simulink model "matlab_control_demo_model_navigation"  (R2022b)
settings: Solver=FixedStepAuto  StartTime=0.0  StopTime=inf  RelTol=1e-3
values from neighbouring files (symbols this model uses):
  waypoints = [ ... (first row only)    [load_quadrotor_simulink_control_model_navigation.m]
libraries: slpidlib x10, sharedutil x2, sharedtransform x2, simulink x2, uavalgslib x1, simulink_extras x1
(part 1 of 2)
settings Model: PacingRate=0.100000  Creator=The MathWorks, Inc.  LastModifiedBy=v-zbraude
settings SolverCC: MaxZcPerStep=1
settings OptimizationCC: DefaultParameterBehavior=Inlined  EnhancedBackFolding=on  PassReuseOutputArgsAs=Individual arguments  ZeroExternalMemoryAtStartup=off  ZeroInternalMemoryAtStartup=off  MaxStackSize=64  OptimizeBlockOrder=speed  DifferentSizesBufferReuse=on  OptimizationCustomize=off  EfficientTunableParamExpr=on
settings DebuggingCC: ParameterTunabilityLossMsg=error
settings HardwareCC: ProdBitPerPointer=32  ProdBitPerSizeT=32  ProdBitPerPtrDiffT=32  ProdLargestAtomicInteger=Long  ProdLargestAtomicFloat=Double  ProdWordSize=32  ProdHWDeviceType=ARM Compatible->ARM Cortex
settings ModelReferenceCC: EnableRefExpFcnMdlSchedulingChecks=on
settings SFSimCC: MATLABDynamicMemAlloc=off
settings RTWCC: Description=Embedded Coder  SystemTargetFile=ert.tlc  TemplateMakefile=ert_default_tmf  Toolchain=GNU Tools for PX4 Autopilots  DLArmComputeVersion=19.05
settings CodeAppCC: ForceParamTrailComments=on  IgnoreCustomStorageClasses=off  MaxIdLength=63  OperatorAnnotations=on  SimulinkDataObjDesc=on  SFDataObjDesc=on  InsertBlockDesc=on
settings ERTTargetCC: ExtModeTransport=3  ExtModeStaticAlloc=on  ExtModeMexFile=ext_xcp  ExtModeIntrfLevel=Level2 - Open  ERTCustomFileTemplate=example_file_process.tlc

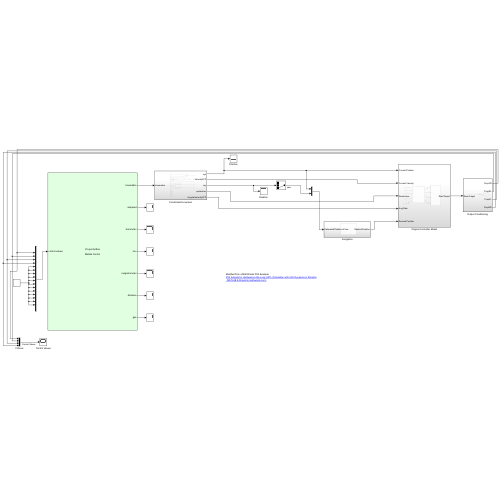
[thumbnail: Simulink's stored preview of the top-level diagram]
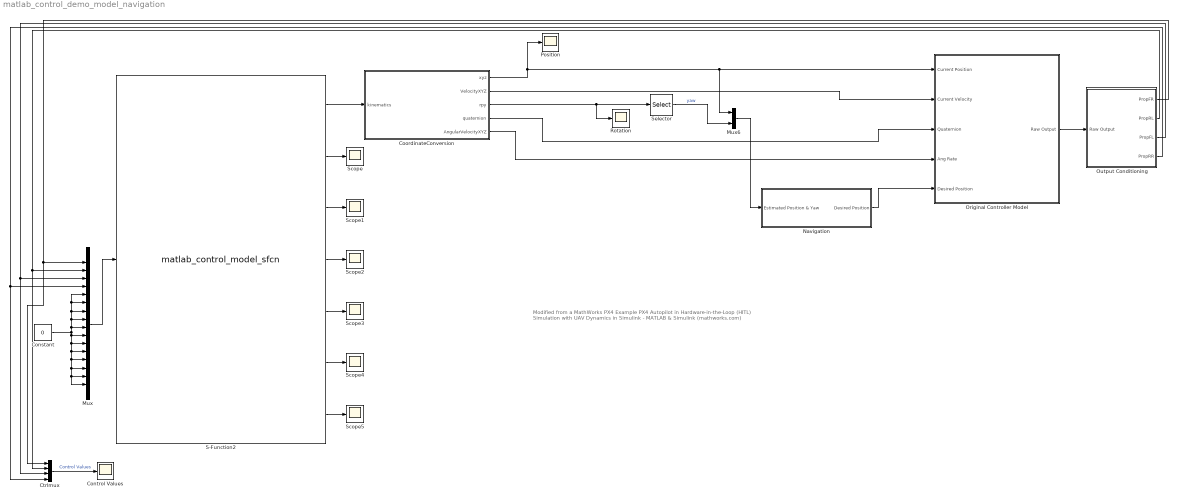
== system matlab_control_demo_model_navigation ==
  note: Modified from a MathWorks PX4 Example
      | PX4 Autopilot in Hardware-in-the-Loop (HITL) Simulation with UAV Dynamics in Simulink - MATLAB & Simulink (mathworks.com)
  Constant : Constant  Value=0
  Control Values : Scope
  CoordinateConversion : Subsystem
  Ctrlmux : Mux
  Mux : Mux  Inputs=16
  Mux6 : Mux  Inputs=2
  Navigation : Subsystem
  Original Controller Model : Subsystem
  Output Conditioning : Subsystem
  Position : Scope
  Rotation : Scope
  S-Function2 : S-Function  Priority=1  FunctionName=matlab_control_model_sfcn  Parameters=hostname,portnumber,timestep  SFunctionDeploymentMode=off  EnableBusSupport=off  mask{hostname=*, portnumber=8998, timestep=0.003}
      mask prompts: hostname "Host name:"; portnumber "Port number:"; timestep "AirSim time step:"
      mask Display:
      | disp("Project AirSim\n\n")
      | disp("\n\nMatlab Control")
      | port_label('input',1,'control values')
      | port_label('output',1,'kinematics')
      | port_label('output',2,'airspeed')
      | port_label('output',3,'barometer')
      | port_label('output',4,'imu')
      | port_label('output',5,'magnetometer')
      | port_label('output',6,'distance')
      | port_label('output',7,'gps')
  Scope{,1..5} (6 alike) : Scope
  Selector : Selector  InputPortWidth=3  IndexOptions=Index vector (dialog)  Indices=[3]  OutputSizes=1
  wires:
  S-Function2/6 -> Scope4/1
  S-Function2/5 -> Scope3/1
  S-Function2/3 -> Scope1/1
  S-Function2/2 -> Scope/1
  Mux/1 -> S-Function2/1
  Constant/1 -> Mux/10, Mux/16, Mux/15, Mux/14, Mux/13, Mux/12, Mux/11, Mux/9, Mux/8, Mux/7, Mux/6, Mux/5
  Ctrlmux/1 -> Control Values/1  "Control Values"
  S-Function2/4 -> Scope2/1
  S-Function2/7 -> Scope5/1
  Mux6/1 -> Navigation/1(Estimated Position & Yaw)
  Selector/1 -> Mux6/2  "yaw"
  CoordinateConversion/1(xyz) -> Position/1, Mux6/1, Original Controller Model/1(Current Position)
  CoordinateConversion/3(rpy) -> Rotation/1, Selector/1
  S-Function2/1 -> CoordinateConversion/1(kinematics)
  CoordinateConversion/2(VelocityXYZ) -> Original Controller Model/2(Current Velocity)
  CoordinateConversion/4(quaternion) -> Original Controller Model/3(Quaternion)
  CoordinateConversion/5(AngularVelocityXYZ) -> Original Controller Model/4(Ang Rate)
  Navigation/1(Desired Position) -> Original Controller Model/5(Desired Position)
  Original Controller Model/1(Raw Output) -> Output Conditioning/1(Raw Output)
  Output Conditioning/1(PropFR) -> Mux/1, Ctrlmux/1
  Output Conditioning/2(PropRL) -> Ctrlmux/2, Mux/2
  Output Conditioning/3(PropFL) -> Ctrlmux/3, Mux/3
  Output Conditioning/4(PropRR) -> Ctrlmux/4, Mux/4

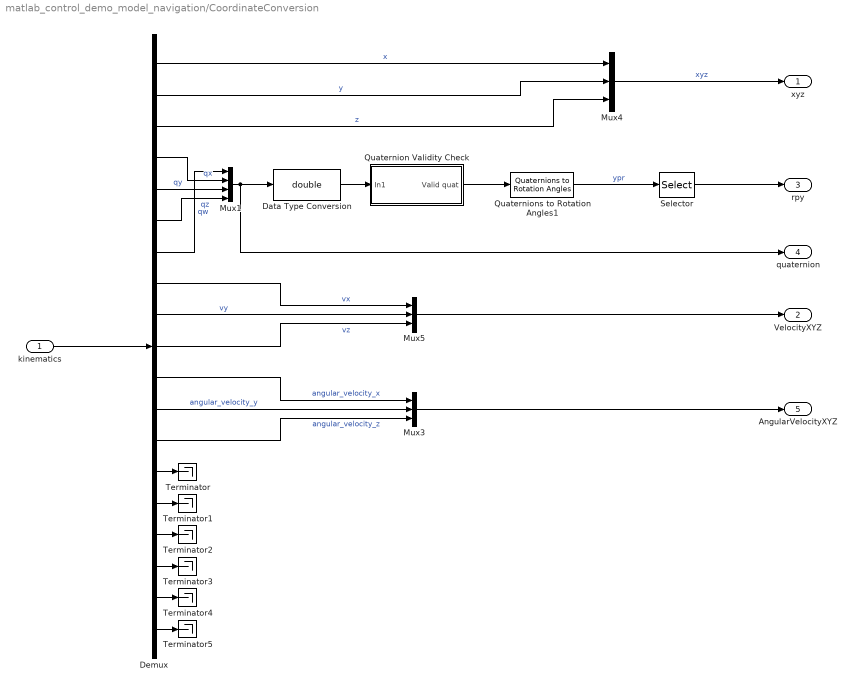
== system matlab_control_demo_model_navigation/CoordinateConversion ==
  kinematics : Inport
  Data Type Conversion : DataTypeConversion  OutDataTypeStr=double  SaturateOnIntegerOverflow=off  RndMeth=Floor
  Demux : Demux  Outputs=19
  Mux1 : Mux
  Mux3 : Mux  Inputs=3
  Mux4 : Mux  Inputs=3
  Mux5 : Mux  Inputs=3
  Quaternion Validity Check : Subsystem
  Quaternions to Rotation Angles1 : sharedtransform/Quaternions to Rotation Angles  rotationOrder=ZYX  aMode=aMode
  Selector : Selector  InputPortWidth=3  IndexOptions=Index vector (dialog)  Indices=[3 2 1]  OutputSizes=1
  Terminator{,1..5} (6 alike) : Terminator
  xyz : Outport
  VelocityXYZ : Outport  Port=2
  rpy : Outport  Port=3
  quaternion : Outport  Port=4
  AngularVelocityXYZ : Outport  Port=5
  wires:
  Mux1/1 -> Data Type Conversion/1, quaternion/1
  Demux/16 -> Terminator2/1
  Demux/1 -> Mux4/1  "x"
  Demux/2 -> Mux4/2  "y"
  Demux/3 -> Mux4/3  "z"
  Demux/14 -> Terminator/1
  Demux/15 -> Terminator1/1
  Mux4/1 -> xyz/1  "xyz"
  Demux/6 -> Mux1/4  "qz"
  Demux/9 -> Mux5/2  "vy"
  Demux/10 -> Mux5/3  "vz"
  Demux/19 -> Terminator5/1
  Demux/5 -> Mux1/3  "qy"
  Demux/13 -> Mux3/3  "angular_velocity_z"
  Demux/7 -> Mux1/1  "qw"
  Demux/12 -> Mux3/2  "angular_velocity_y"
  Demux/8 -> Mux5/1  "vx"
  Demux/4 -> Mux1/2  "qx"
  Demux/11 -> Mux3/1  "angular_velocity_x"
  Demux/18 -> Terminator4/1
  kinematics/1 -> Demux/1
  Mux5/1 -> VelocityXYZ/1
  Demux/17 -> Terminator3/1
  Mux3/1 -> AngularVelocityXYZ/1
  Data Type Conversion/1 -> Quaternion Validity Check/1(In1)
  Quaternion Validity Check/1(Valid quat) -> Quaternions to Rotation Angles1/1
  Quaternions to Rotation Angles1/1 -> Selector/1  "ypr"
  Selector/1 -> rpy/1

== system matlab_control_demo_model_navigation/Navigation ==
  Estimated Position & Yaw : Inport
  Quadcopter Navigation Algorithm : Subsystem  Variant=on
  Desired Position : Outport
  wires:
  Quadcopter Navigation Algorithm/1(Desired Position) -> Desired Position/1
  Estimated Position & Yaw/1 -> Quadcopter Navigation Algorithm/1(Current Position)

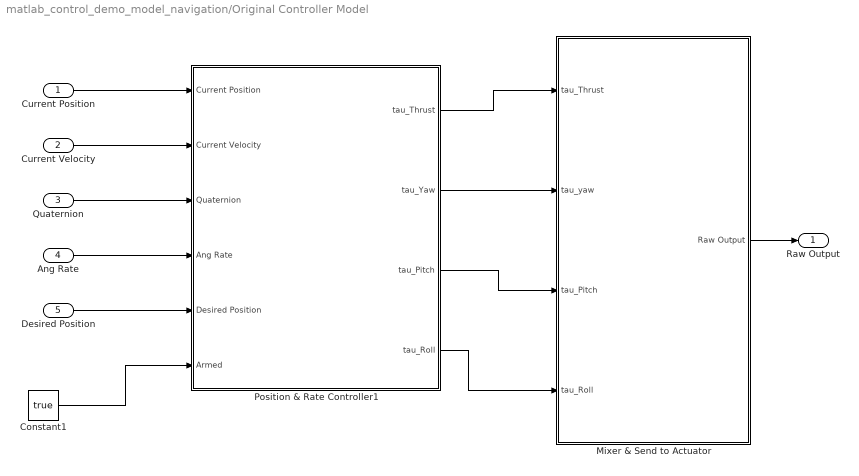
== system matlab_control_demo_model_navigation/Original Controller Model ==
  Current Position : Inport
  Current Velocity : Inport  Port=2
  Quaternion : Inport  Port=3
  Ang Rate : Inport  Port=4
  Desired Position : Inport  Port=5
  Constant1 : Constant  Value=true
  Mixer & Send to Actuator : Subsystem
  Position & Rate Controller1 : Subsystem
  Raw Output : Outport
  wires:
  Constant1/1 -> Position & Rate Controller1/6(Armed)
  Position & Rate Controller1/1(tau_Thrust) -> Mixer & Send to Actuator/1(tau_Thrust)
  Position & Rate Controller1/2(tau_Yaw) -> Mixer & Send to Actuator/2(tau_yaw)
  Position & Rate Controller1/3(tau_Pitch) -> Mixer & Send to Actuator/3(tau_Pitch)
  Position & Rate Controller1/4("tau_Roll ") -> Mixer & Send to Actuator/4(tau_Roll)
  Mixer & Send to Actuator/1(Raw Output) -> Raw Output/1
  Current Position/1 -> Position & Rate Controller1/1(Current Position)
  Current Velocity/1 -> Position & Rate Controller1/2(Current Velocity)
  Quaternion/1 -> Position & Rate Controller1/3(Quaternion)
  Ang Rate/1 -> Position & Rate Controller1/4(Ang Rate)
  Desired Position/1 -> Position & Rate Controller1/5(Desired Position)

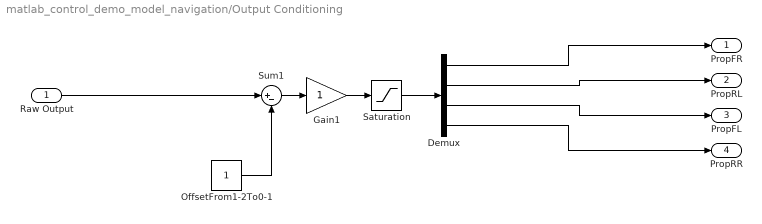
== system matlab_control_demo_model_navigation/Output Conditioning ==
  Raw Output : Inport
  Demux : Demux
  Gain1 : Gain  OutDataTypeStr=double
  OffsetFrom1-2To0-1 : Constant
  Saturation : Saturate  UpperLimit=1  LowerLimit=0
  Sum1 : Sum  Inputs=|+-
  PropFR : Outport
  PropRL : Outport  Port=2
  PropFL : Outport  Port=3
  PropRR : Outport  Port=4
  wires:
  OffsetFrom1-2To0-1/1 -> Sum1/2
  Demux/2 -> PropRL/1
  Demux/4 -> PropRR/1
  Demux/1 -> PropFR/1
  Gain1/1 -> Saturation/1
  Demux/3 -> PropFL/1
  Saturation/1 -> Demux/1
  Sum1/1 -> Gain1/1
  Raw Output/1 -> Sum1/1

== system matlab_control_demo_model_navigation/CoordinateConversion/Quaternion Validity Check ==
  In1 : Inport
  Constant : Constant  Value=[1 0 0 0]  SampleTime=-1
  Quaternion Norm : sharedutil/Quaternion Norm  aMode=aMode
  Switch : Switch  Criteria=u2 > Threshold  SaturateOnIntegerOverflow=off  InputSameDT=off
  Valid quat : Outport
  wires:
  In1/1 -> Quaternion Norm/1, Switch/1
  Quaternion Norm/1 -> Switch/2
  Switch/1 -> Valid quat/1
  Constant/1 -> Switch/3

== system matlab_control_demo_model_navigation/Navigation/Quadcopter Navigation Algorithm ==
  Current Position : Inport
  Manual Waypoints : Subsystem  VariantControl=guidanceType == 1
  Manual Waypoints from Simulink Dashboard : Subsystem  VariantControl=guidanceType == 2
  Desired Position : Outport

== system matlab_control_demo_model_navigation/Original Controller Model/Mixer & Send to Actuator ==
  tau_Thrust : Inport
  tau_yaw : Inport  Port=2
  tau_Pitch : Inport  Port=3
  tau_Roll : Inport  Port=4
  Mixer matrix : Constant  Value=[1 -1 1 1;1 1 -1 1;1 -1 -1 -1;1 1 1 -1]  OutDataTypeStr=Inherit: Inherit via back propagation  SampleTime=-1
  Mux2 : Mux
  Product2 : Product  Multiplication=Matrix(*)  RndMeth=Zero
  Raw Output : Outport
  wires:
  Mux2/1 -> Product2/2
  tau_Roll/1 -> Mux2/3  "roll_cmd"
  tau_Thrust/1 -> Mux2/1  "thrust cmd"
  tau_yaw/1 -> Mux2/4
  Mixer matrix/1 -> Product2/1
  tau_Pitch/1 -> Mux2/2  "pitch cmd"
  Product2/1 -> Raw Output/1

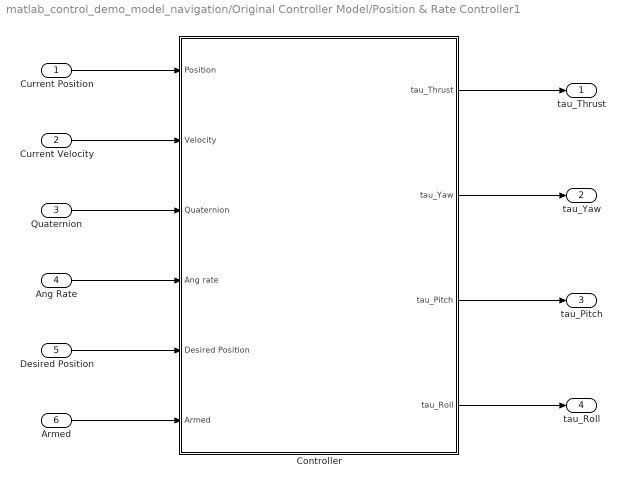
== system matlab_control_demo_model_navigation/Original Controller Model/Position & Rate Controller1 ==
  Current Position : Inport
  Current Velocity : Inport  Port=2
  Quaternion : Inport  Port=3
  Ang Rate : Inport  Port=4
  Desired Position : Inport  Port=5
  Armed : Inport  Port=6
  Controller : Subsystem
  tau_Thrust : Outport
  tau_Yaw : Outport  Port=2
  tau_Pitch : Outport  Port=3
  "tau_Roll " : Outport  Port=4
  wires:
  Controller/3(tau_Pitch) -> tau_Pitch/1
  Quaternion/1 -> Controller/3(Quaternion)
  Controller/2(tau_Yaw) -> tau_Yaw/1
  Controller/4("tau_Roll ") -> "tau_Roll "/1
  Current Velocity/1 -> Controller/2(Velocity)
  Current Position/1 -> Controller/1(Position)
  Controller/1(tau_Thrust) -> tau_Thrust/1
  Desired Position/1 -> Controller/5(Desired Position)
  Ang Rate/1 -> Controller/4(Ang rate)
  Armed/1 -> Controller/6(Armed)

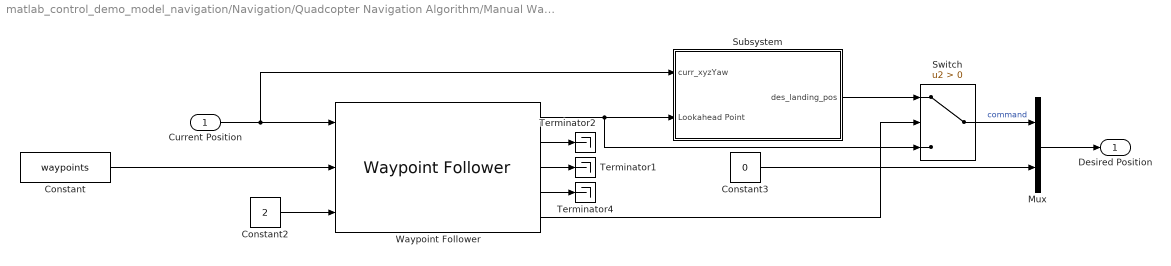
== system matlab_control_demo_model_navigation/Navigation/Quadcopter Navigation Algorithm/Manual Waypoints ==
  Current Position : Inport
  Constant : Constant  Value=waypoints
  Constant2 : Constant  Value=2  SampleTime=-1
  Constant3 : Constant  Value=0  SampleTime=-1
  Mux : Mux  Inputs=2
  Subsystem : Subsystem
  Switch : Switch  Criteria=u2 > Threshold  SaturateOnIntegerOverflow=off  InputSameDT=off
  Terminator1 : Terminator
  Terminator2 : Terminator
  Terminator4 : Terminator
  Waypoint Follower : uavalgslib/Waypoint Follower  UAVType=multirotor  StartFrom=first  TransitionRadiusSource=internal  TransitionRadius=5  MinLookaheadDistance=0.1  YawInput=on  ShowCrossTrackErrorOutput=off  ShowStatusOutput=on  SimulateUsing=Interpreted execution
  Desired Position : Outport
  wires:
  Waypoint Follower/1 -> Subsystem/2(Lookahead Point), Switch/3
  Waypoint Follower/4 -> Terminator4/1
  Subsystem/1(des_landing_pos) -> Switch/1
  Current Position/1 -> Waypoint Follower/1, Subsystem/1(curr_xyzYaw)
  Waypoint Follower/5 -> Switch/2
  Constant2/1 -> Waypoint Follower/3
  Waypoint Follower/2 -> Terminator2/1
  Switch/1 -> Mux/1  "command"
  Mux/1 -> Desired Position/1
  Waypoint Follower/3 -> Terminator1/1
  Constant3/1 -> Mux/2
  Constant/1 -> Waypoint Follower/2

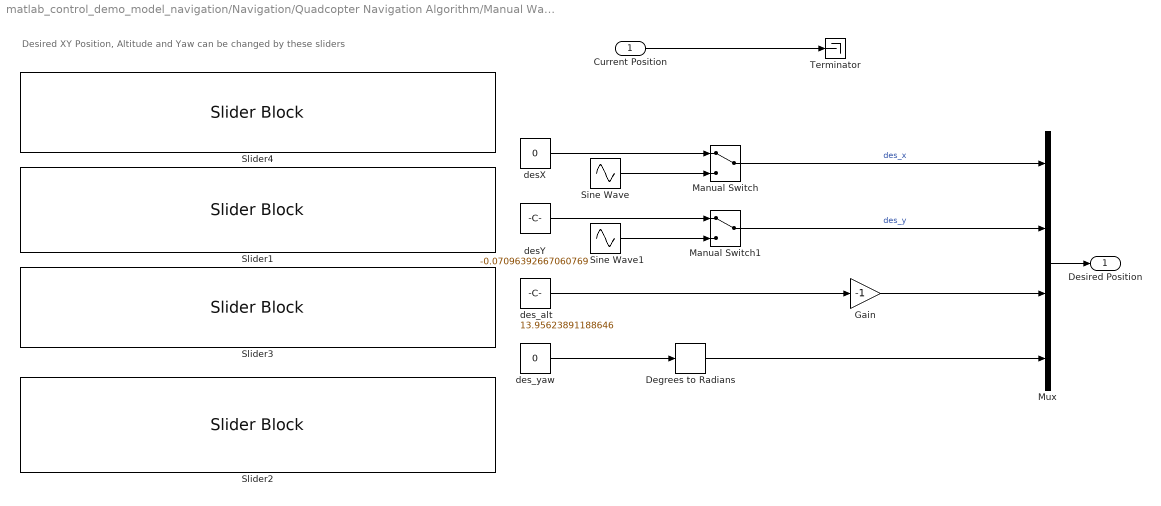
== system matlab_control_demo_model_navigation/Navigation/Quadcopter Navigation Algorithm/Manual Waypoints from Simulink Dashboard ==
  note: Desired XY Position, Altitude and Yaw can be changed by these sliders
  Current Position : Inport  PortDimensions=[1 4]
  Degrees to Radians : simulink_extras/Transformations/Degrees to Radians
  Gain : Gain  Gain=-1
  Manual Switch : ManualSwitch
  Manual Switch1 : ManualSwitch
  Mux : Mux
  Sine Wave : Sin  Amplitude=80  Frequency=2*pi*0.005
  Sine Wave1 : Sin  Amplitude=80  Frequency=2*pi*0.005  Phase=pi/2
  Slider1 : SliderBlock  ScaleMin=-20  ScaleMax=20  TickInterval=2
  Slider2 : SliderBlock  ScaleMin=-180  ScaleMax=180
  Slider3 : SliderBlock
  Slider4 : SliderBlock  ScaleMin=-20  ScaleMax=20  TickInterval=2
  Terminator : Terminator
  desX : Constant  Value=0  SampleTime=-1
  desY : Constant  Value=-0.07096392667060769  SampleTime=-1
  des_alt : Constant  Value=13.95623891188646  SampleTime=-1
  des_yaw : Constant  Value=0  SampleTime=-1
  Desired Position : Outport
  wires:
  desY/1 -> Manual Switch1/1
  Sine Wave/1 -> Manual Switch/2
  desX/1 -> Manual Switch/1
  Manual Switch1/1 -> Mux/2  "des_y"
  des_yaw/1 -> Degrees to Radians/1
  Manual Switch/1 -> Mux/1  "des_x"
  Sine Wave1/1 -> Manual Switch1/2
  Mux/1 -> Desired Position/1
  Current Position/1 -> Terminator/1
  des_alt/1 -> Gain/1
  Degrees to Radians/1 -> Mux/4
  Gain/1 -> Mux/3

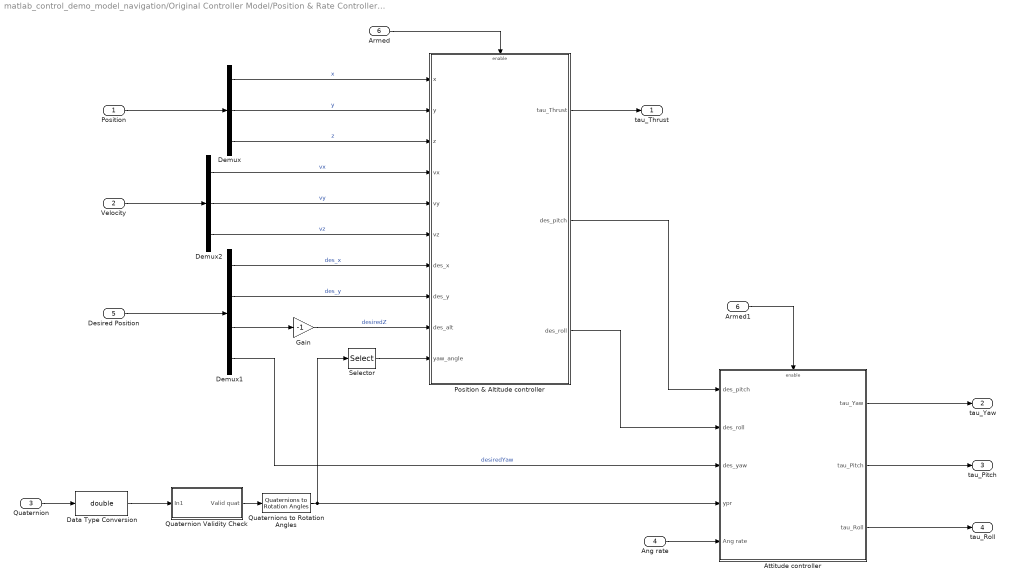
== system matlab_control_demo_model_navigation/Original Controller Model/Position & Rate Controller1/Controller ==
  Position : Inport
  Velocity : Inport  Port=2
  Quaternion : Inport  Port=3
  Ang rate : Inport  Port=4
  Desired Position : Inport  Port=5
  Armed : Inport  Port=6
  Armed1 : InportShadow  Port=6
  Attitude controller : Subsystem
  Data Type Conversion : DataTypeConversion  OutDataTypeStr=double  SaturateOnIntegerOverflow=off  RndMeth=Floor
  Demux : Demux  Outputs=3
  Demux1 : Demux
  Demux2 : Demux  Outputs=3
  Gain : Gain  Gain=-1
  Position & Altitude controller : Subsystem
  Quaternion Validity Check : Subsystem
  Quaternions to Rotation Angles : sharedtransform/Quaternions to Rotation Angles  rotationOrder=ZYX  aMode=aMode
  Selector : Selector  InputPortWidth=3  IndexOptions=Index vector (dialog)  Indices=[1]  OutputSizes=1
  tau_Thrust : Outport
  tau_Yaw : Outport  Port=2
  tau_Pitch : Outport  Port=3
  "tau_Roll " : Outport  Port=4
  wires:
  Attitude controller/3(tau_Roll) -> "tau_Roll "/1
  Attitude controller/2(tau_Pitch) -> tau_Pitch/1
  Attitude controller/1(tau_Yaw) -> tau_Yaw/1
  Position & Altitude controller/2(des_pitch) -> Attitude controller/1(des_pitch)
  Position & Altitude controller/3(des_roll) -> Attitude controller/2(des_roll)
  Demux/2 -> Position & Altitude controller/2(y)  "y"
  Gain/1 -> Position & Altitude controller/9(des_alt)  "desiredZ"
  Demux2/2 -> Position & Altitude controller/5(vy)  "vy"
  Demux1/1 -> Position & Altitude controller/7(des_x)  "des_x"
  Demux2/1 -> Position & Altitude controller/4(vx)  "vx"
  Demux1/3 -> Gain/1
  Demux/1 -> Position & Altitude controller/1(x)  "x"
  Demux1/2 -> Position & Altitude controller/8(des_y)  "des_y"
  Position & Altitude controller/1(tau_Thrust) -> tau_Thrust/1
  Desired Position/1 -> Demux1/1
  Demux2/3 -> Position & Altitude controller/6(vz)  "vz"
  Demux/3 -> Position & Altitude controller/3(z)  "z"
  Quaternion/1 -> Data Type Conversion/1
  Data Type Conversion/1 -> Quaternion Validity Check/1(In1)
  Position/1 -> Demux/1
  Velocity/1 -> Demux2/1
  Quaternion Validity Check/1(Valid quat) -> Quaternions to Rotation Angles/1
  Ang rate/1 -> Attitude controller/5(Ang rate)
  Quaternions to Rotation Angles/1 -> Selector/1, Attitude controller/4(ypr)
  Selector/1 -> Position & Altitude controller/10(yaw_angle)
  Demux1/4 -> Attitude controller/3(des_yaw)  "desiredYaw"
  Armed/1 -> Position & Altitude controller/Enable
  Armed1/1 -> Attitude controller/Enable

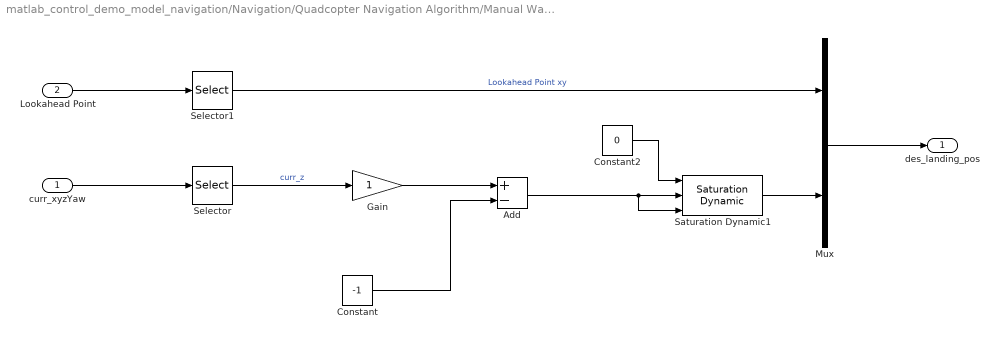
== system matlab_control_demo_model_navigation/Navigation/Quadcopter Navigation Algorithm/Manual Waypoints/Subsystem ==
  curr_xyzYaw : Inport
  Lookahead Point : Inport  Port=2
  Add : Sum  Inputs=+-
  Constant : Constant  Value=-1  OutDataTypeStr=Inherit: Inherit via back propagation
  Constant2 : Constant  Value=0  OutDataTypeStr=Inherit: Inherit via back propagation
  Gain : Gain
  Mux : Mux  Inputs=2
  Saturation Dynamic1 : simulink/Discontinuities/Saturation Dynamic  OutMin=0  OutMax=[]  OutDataTypeStr=Inherit: Same as second input  OutDataType=fixdt(1, 16)  OutScaling=2^-10  DoSatur=off
  Selector : Selector  InputPortWidth=4  IndexOptions=Index vector (dialog)  Indices=[3]  OutputSizes=1
  Selector1 : Selector  InputPortWidth=3  IndexOptions=Index vector (dialog)  Indices=[1 2]  OutputSizes=1
  des_landing_pos : Outport
  wires:
  Gain/1 -> Add/1
  Constant/1 -> Add/2
  Mux/1 -> des_landing_pos/1
  curr_xyzYaw/1 -> Selector/1
  Selector/1 -> Gain/1  "curr_z"
  Lookahead Point/1 -> Selector1/1
  Selector1/1 -> Mux/1  "Lookahead Point xy"
  Constant2/1 -> Saturation Dynamic1/1
  Add/1 -> Saturation Dynamic1/2, Saturation Dynamic1/3
  Saturation Dynamic1/1 -> Mux/2

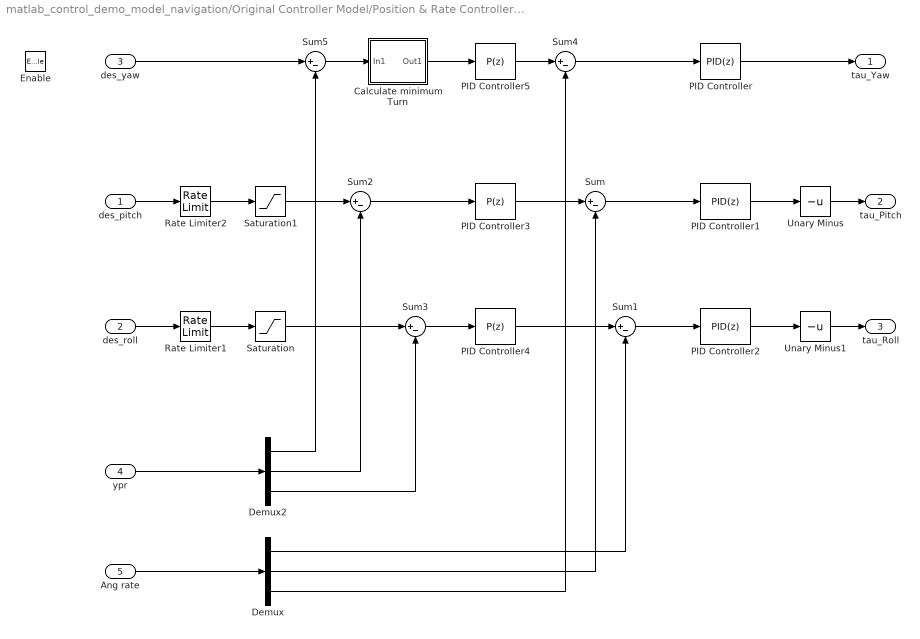
== system matlab_control_demo_model_navigation/Original Controller Model/Position & Rate Controller1/Controller/Attitude controller ==
  des_pitch : Inport
  des_roll : Inport  Port=2
  des_yaw : Inport  Port=3
  ypr : Inport  Port=4
  Ang rate : Inport  Port=5
  Enable : EnablePort
  Calculate minimum Turn : Subsystem
  Demux : Demux  Outputs=3
  Demux2 : Demux  Outputs=3
  PID Controller : slpidlib/PID Controller  Controller=PID  Form=Parallel  TimeDomain=Discrete-time  UseExternalTs=off  SampleTime=-1  IntegratorMethod=Forward Euler  FilterMethod=Forward Euler  ControllerParametersSource=internal  P=0.2  I=0  UseKiTs=off  D=0  N=100  UseFilter=on  TunerSelectOption=Transfer Function Based (PID Tuner App)  InitialConditionSource=internal  InitialConditionForIntegrator=0  InitialConditionForFilter=0  DifferentiatorICPrevScaledInput=0  ExternalReset=none  TrackingMode=off  Kt=1  LimitOutput=on  SatLimitsSource=internal  UpperSaturationLimit=0.1  LowerSaturationLimit=-0.1  LinearizeAsGain=on  AntiWindupMode=clamping  Kb=1  LimitIntegrator=off  UpperIntegratorSaturationLimit=inf  LowerIntegratorSaturationLimit=-inf  POutMin=[]  POutMax=[]  IOutMin=[]  IOutMax=[]  DOutMin=[]  DOutMax=[]  NOutMin=[]  NOutMax=[]  SumOutMin=[]  SumOutMax=[]  SaturationOutMin=[]  SaturationOutMax=[]  PParamMin=[]  PParamMax=[]  IParamMin=[]  IParamMax=[]  DParamMin=[]  DParamMax=[]  NParamMin=[]  NParamMax=[]  KbParamMin=[]  KbParamMax=[]  KtParamMin=[]  KtParamMax=[]  KbOutMin=[]  KbOutMax=[]  KtOutMin=[]  KtOutMax=[]  IntegratorOutMin=[]  IntegratorOutMax=[]  FilterOutMin=[]  FilterOutMax=[]  SumI1OutMin=[]  SumI1OutMax=[]  SumI2OutMin=[]  SumI2OutMax=[]  SumI3OutMin=[]  SumI3OutMax=[]  SumI4OutMin=[]  SumI4OutMax=[]  SumDOutMin=[]  SumDOutMax=[]  DifferentiatorOutMin=[]  DifferentiatorOutMax=[]  FilterDiffOutCoefMin=[]  FilterDiffOutCoefMax=[]  ReciprocalOutMin=[]  ReciprocalOutMax=[]  SumDenOutMin=[]  SumDenOutMax=[]  SumNumOutMin=[]  SumNumOutMax=[]  DivideOutMin=[]  DivideOutMax=[]  UdiffTsProdOutMin=[]  UdiffTsProdOutMax=[]  NTsProdOutMin=[]  NTsProdOutMax=[]  UintegralTsProdOutMin=[]  UintegralTsProdOutMax=[]  UngainTsProdOutMin=[]  UngainTsProdOutMax=[]  ClampingZeroOutDataTypeStr=Inherit: Inherit via back propagation  ClampingZeroOutMin=[]  ClampingZeroOutMax=[]  FilterDenConstantOutDataTypeStr=Inherit: Inherit via back propagation  FilterDenConstantOutMin=[]  FilterDenConstantOutMax=[]  PCopyOutDataTypeStr=Inherit: Inherit via back propagation  PCopyOutMin=[]  PCopyOutMax=[]  NCopyOutDataTypeStr=Inherit: Inherit via back propagation  NCopyOutMin=[]  NCopyOutMax=[]  IntegratorContinuousStateAttributes=''  IntegratorStateMustResolveToSignalObject=off  IntegratorRTWStateStorageClass=Auto  FilterContinuousStateAttributes=''  FilterStateMustResolveToSignalObject=off  FilterRTWStateStorageClass=Auto  ParallelPVariant=InternalParameters  IdealPVariant=Disabled  IVariant=InternalParameters  DVariant=InternalParameters  IntegratorVariant=Discrete  SatVariant=Enabled  AWVariant=DiscClampingParallel  PCopyVariant=Disabled  TRVariant=Disabled  FdbkBlocksVariant=Forward  IdealPFdbkVariant=Disabled  SatFdbkVariant=Disabled  DerivativeFilterVariant=ForwardEulerFilter  NVariant=InternalParameters  NCopyVariant=Disabled  FilterICVariant=InternalICsFilter  IntegratorICVariant=InternalICs  ExternalResetVariant=Disabled  TRSumVariant=Passthrough  SumFdbkVariant=Disabled  SumVariant=Sum_PID  TsampFilterVariant=InternalTs  TsampNgainVariant=Passthrough  TsampIntegralVariant=Passthrough  ExternalSaturationOutDataTypeStr=Inherit: Same as second input
  PID Controller1 : slpidlib/PID Controller  Controller=PID  Form=Parallel  TimeDomain=Discrete-time  UseExternalTs=off  SampleTime=-1  IntegratorMethod=Forward Euler  FilterMethod=Forward Euler  ControllerParametersSource=internal  P=0.035  I=0  UseKiTs=off  D=0.05/20  N=50  UseFilter=on  TunerSelectOption=Transfer Function Based (PID Tuner App)  InitialConditionSource=internal  InitialConditionForIntegrator=0  InitialConditionForFilter=0  DifferentiatorICPrevScaledInput=0  ExternalReset=none  TrackingMode=off  Kt=1  LimitOutput=on  SatLimitsSource=internal  UpperSaturationLimit=0.2  LowerSaturationLimit=-0.2  LinearizeAsGain=on  AntiWindupMode=clamping  Kb=1  LimitIntegrator=off  UpperIntegratorSaturationLimit=inf  LowerIntegratorSaturationLimit=-inf  POutMin=[]  POutMax=[]  IOutMin=[]  IOutMax=[]  DOutMin=[]  DOutMax=[]  NOutMin=[]  NOutMax=[]  SumOutMin=[]  SumOutMax=[]  SaturationOutMin=[]  SaturationOutMax=[]  PParamMin=[]  PParamMax=[]  IParamMin=[]  IParamMax=[]  DParamMin=[]  DParamMax=[]  NParamMin=[]  NParamMax=[]  KbParamMin=[]  KbParamMax=[]  KtParamMin=[]  KtParamMax=[]  KbOutMin=[]  KbOutMax=[]  KtOutMin=[]  KtOutMax=[]  IntegratorOutMin=[]  IntegratorOutMax=[]  FilterOutMin=[]  FilterOutMax=[]  SumI1OutMin=[]  SumI1OutMax=[]  SumI2OutMin=[]  SumI2OutMax=[]  SumI3OutMin=[]  SumI3OutMax=[]  SumI4OutMin=[]  SumI4OutMax=[]  SumDOutMin=[]  SumDOutMax=[]  DifferentiatorOutMin=[]  DifferentiatorOutMax=[]  FilterDiffOutCoefMin=[]  FilterDiffOutCoefMax=[]  ReciprocalOutMin=[]  ReciprocalOutMax=[]  SumDenOutMin=[]  SumDenOutMax=[]  SumNumOutMin=[]  SumNumOutMax=[]  DivideOutMin=[]  DivideOutMax=[]  UdiffTsProdOutMin=[]  UdiffTsProdOutMax=[]  NTsProdOutMin=[]  NTsProdOutMax=[]  UintegralTsProdOutMin=[]  UintegralTsProdOutMax=[]  UngainTsProdOutMin=[]  UngainTsProdOutMax=[]  ClampingZeroOutDataTypeStr=Inherit: Inherit via back propagation  ClampingZeroOutMin=[]  ClampingZeroOutMax=[]  FilterDenConstantOutDataTypeStr=Inherit: Inherit via back propagation  FilterDenConstantOutMin=[]  FilterDenConstantOutMax=[]  PCopyOutDataTypeStr=Inherit: Inherit via back propagation  PCopyOutMin=[]  PCopyOutMax=[]  NCopyOutDataTypeStr=Inherit: Inherit via back propagation  NCopyOutMin=[]  NCopyOutMax=[]  IntegratorContinuousStateAttributes=''  IntegratorStateMustResolveToSignalObject=off  IntegratorRTWStateStorageClass=Auto  FilterContinuousStateAttributes=''  FilterStateMustResolveToSignalObject=off  FilterRTWStateStorageClass=Auto  ParallelPVariant=InternalParameters  IdealPVariant=Disabled  IVariant=InternalParameters  DVariant=InternalParameters  IntegratorVariant=Discrete  SatVariant=Enabled  AWVariant=DiscClampingParallel  PCopyVariant=Disabled  TRVariant=Disabled  FdbkBlocksVariant=Forward  IdealPFdbkVariant=Disabled  SatFdbkVariant=Disabled  DerivativeFilterVariant=ForwardEulerFilter  NVariant=InternalParameters  NCopyVariant=Disabled  FilterICVariant=InternalICsFilter  IntegratorICVariant=InternalICs  ExternalResetVariant=Disabled  TRSumVariant=Passthrough  SumFdbkVariant=Disabled  SumVariant=Sum_PID  TsampFilterVariant=InternalTs  TsampNgainVariant=Passthrough  TsampIntegralVariant=Passthrough  ExternalSaturationOutDataTypeStr=Inherit: Same as second input
  PID Controller2 : slpidlib/PID Controller  Controller=PID  Form=Parallel  TimeDomain=Discrete-time  UseExternalTs=off  SampleTime=-1  IntegratorMethod=Forward Euler  FilterMethod=Forward Euler  ControllerParametersSource=internal  P=0.035  I=0  UseKiTs=off  D=0.05/20  N=50  UseFilter=on  TunerSelectOption=Transfer Function Based (PID Tuner App)  InitialConditionSource=internal  InitialConditionForIntegrator=0  InitialConditionForFilter=0  DifferentiatorICPrevScaledInput=0  ExternalReset=none  TrackingMode=off  Kt=1  LimitOutput=on  SatLimitsSource=internal  UpperSaturationLimit=0.2  LowerSaturationLimit=-0.2  LinearizeAsGain=on  AntiWindupMode=clamping  Kb=1  LimitIntegrator=off  UpperIntegratorSaturationLimit=inf  LowerIntegratorSaturationLimit=-inf  POutMin=[]  POutMax=[]  IOutMin=[]  IOutMax=[]  DOutMin=[]  DOutMax=[]  NOutMin=[]  NOutMax=[]  SumOutMin=[]  SumOutMax=[]  SaturationOutMin=[]  SaturationOutMax=[]  PParamMin=[]  PParamMax=[]  IParamMin=[]  IParamMax=[]  DParamMin=[]  DParamMax=[]  NParamMin=[]  NParamMax=[]  KbParamMin=[]  KbParamMax=[]  KtParamMin=[]  KtParamMax=[]  KbOutMin=[]  KbOutMax=[]  KtOutMin=[]  KtOutMax=[]  IntegratorOutMin=[]  IntegratorOutMax=[]  FilterOutMin=[]  FilterOutMax=[]  SumI1OutMin=[]  SumI1OutMax=[]  SumI2OutMin=[]  SumI2OutMax=[]  SumI3OutMin=[]  SumI3OutMax=[]  SumI4OutMin=[]  SumI4OutMax=[]  SumDOutMin=[]  SumDOutMax=[]  DifferentiatorOutMin=[]  DifferentiatorOutMax=[]  FilterDiffOutCoefMin=[]  FilterDiffOutCoefMax=[]  ReciprocalOutMin=[]  ReciprocalOutMax=[]  SumDenOutMin=[]  SumDenOutMax=[]  SumNumOutMin=[]  SumNumOutMax=[]  DivideOutMin=[]  DivideOutMax=[]  UdiffTsProdOutMin=[]  UdiffTsProdOutMax=[]  NTsProdOutMin=[]  NTsProdOutMax=[]  UintegralTsProdOutMin=[]  UintegralTsProdOutMax=[]  UngainTsProdOutMin=[]  UngainTsProdOutMax=[]  ClampingZeroOutDataTypeStr=Inherit: Inherit via back propagation  ClampingZeroOutMin=[]  ClampingZeroOutMax=[]  FilterDenConstantOutDataTypeStr=Inherit: Inherit via back propagation  FilterDenConstantOutMin=[]  FilterDenConstantOutMax=[]  PCopyOutDataTypeStr=Inherit: Inherit via back propagation  PCopyOutMin=[]  PCopyOutMax=[]  NCopyOutDataTypeStr=Inherit: Inherit via back propagation  NCopyOutMin=[]  NCopyOutMax=[]  IntegratorContinuousStateAttributes=''  IntegratorStateMustResolveToSignalObject=off  IntegratorRTWStateStorageClass=Auto  FilterContinuousStateAttributes=''  FilterStateMustResolveToSignalObject=off  FilterRTWStateStorageClass=Auto  ParallelPVariant=InternalParameters  IdealPVariant=Disabled  IVariant=InternalParameters  DVariant=InternalParameters  IntegratorVariant=Discrete  SatVariant=Enabled  AWVariant=DiscClampingParallel  PCopyVariant=Disabled  TRVariant=Disabled  FdbkBlocksVariant=Forward  IdealPFdbkVariant=Disabled  SatFdbkVariant=Disabled  DerivativeFilterVariant=ForwardEulerFilter  NVariant=InternalParameters  NCopyVariant=Disabled  FilterICVariant=InternalICsFilter  IntegratorICVariant=InternalICs  ExternalResetVariant=Disabled  TRSumVariant=Passthrough  SumFdbkVariant=Disabled  SumVariant=Sum_PID  TsampFilterVariant=InternalTs  TsampNgainVariant=Passthrough  TsampIntegralVariant=Passthrough  ExternalSaturationOutDataTypeStr=Inherit: Same as second input
  PID Controller3 : slpidlib/PID Controller  Controller=P  Form=Parallel  TimeDomain=Discrete-time  UseExternalTs=off  SampleTime=-1  IntegratorMethod=Forward Euler  FilterMethod=Forward Euler  ControllerParametersSource=internal  P=4  I=1  UseKiTs=off  D=0  N=100  UseFilter=on  TunerSelectOption=Transfer Function Based (PID Tuner App)  InitialConditionSource=internal  InitialConditionForIntegrator=0  InitialConditionForFilter=0  DifferentiatorICPrevScaledInput=0  ExternalReset=none  TrackingMode=off  Kt=1  LimitOutput=off  SatLimitsSource=internal  UpperSaturationLimit=inf  LowerSaturationLimit=-inf  LinearizeAsGain=on  AntiWindupMode=none  Kb=1  LimitIntegrator=off  UpperIntegratorSaturationLimit=inf  LowerIntegratorSaturationLimit=-inf  POutMin=[]  POutMax=[]  IOutMin=[]  IOutMax=[]  DOutMin=[]  DOutMax=[]  NOutMin=[]  NOutMax=[]  SumOutMin=[]  SumOutMax=[]  SaturationOutMin=[]  SaturationOutMax=[]  PParamMin=[]  PParamMax=[]  IParamMin=[]  IParamMax=[]  DParamMin=[]  DParamMax=[]  NParamMin=[]  NParamMax=[]  KbParamMin=[]  KbParamMax=[]  KtParamMin=[]  KtParamMax=[]  KbOutMin=[]  KbOutMax=[]  KtOutMin=[]  KtOutMax=[]  IntegratorOutMin=[]  IntegratorOutMax=[]  FilterOutMin=[]  FilterOutMax=[]  SumI1OutMin=[]  SumI1OutMax=[]  SumI2OutMin=[]  SumI2OutMax=[]  SumI3OutMin=[]  SumI3OutMax=[]  SumI4OutMin=[]  SumI4OutMax=[]  SumDOutMin=[]  SumDOutMax=[]  DifferentiatorOutMin=[]  DifferentiatorOutMax=[]  FilterDiffOutCoefMin=[]  FilterDiffOutCoefMax=[]  ReciprocalOutMin=[]  ReciprocalOutMax=[]  SumDenOutMin=[]  SumDenOutMax=[]  SumNumOutMin=[]  SumNumOutMax=[]  DivideOutMin=[]  DivideOutMax=[]  UdiffTsProdOutMin=[]  UdiffTsProdOutMax=[]  NTsProdOutMin=[]  NTsProdOutMax=[]  UintegralTsProdOutMin=[]  UintegralTsProdOutMax=[]  UngainTsProdOutMin=[]  UngainTsProdOutMax=[]  ClampingZeroOutDataTypeStr=Inherit: Inherit via back propagation  ClampingZeroOutMin=[]  ClampingZeroOutMax=[]  FilterDenConstantOutDataTypeStr=Inherit: Inherit via back propagation  FilterDenConstantOutMin=[]  FilterDenConstantOutMax=[]  PCopyOutDataTypeStr=Inherit: Inherit via back propagation  PCopyOutMin=[]  PCopyOutMax=[]  NCopyOutDataTypeStr=Inherit: Inherit via back propagation  NCopyOutMin=[]  NCopyOutMax=[]  IntegratorContinuousStateAttributes=''  IntegratorStateMustResolveToSignalObject=off  IntegratorRTWStateStorageClass=Auto  FilterContinuousStateAttributes=''  FilterStateMustResolveToSignalObject=off  FilterRTWStateStorageClass=Auto  ParallelPVariant=InternalParameters  IdealPVariant=Disabled  IVariant=Disabled  DVariant=Disabled  IntegratorVariant=Disabled  SatVariant=Disabled  AWVariant=Disabled  PCopyVariant=Disabled  TRVariant=Disabled  FdbkBlocksVariant=Forward  IdealPFdbkVariant=Disabled  SatFdbkVariant=Disabled  DerivativeFilterVariant=Disabled  NVariant=Disabled  NCopyVariant=Disabled_SignalSpec  FilterICVariant=Disabled  IntegratorICVariant=Disabled  ExternalResetVariant=Disabled  TRSumVariant=Passthrough  SumFdbkVariant=Disabled  SumVariant=Passthrough_P  TsampFilterVariant=InternalTs  TsampNgainVariant=Passthrough  TsampIntegralVariant=Disabled_SignalSpec  ExternalSaturationOutDataTypeStr=Inherit: Same as second input
  PID Controller4 : slpidlib/PID Controller  Controller=P  Form=Parallel  TimeDomain=Discrete-time  UseExternalTs=off  SampleTime=-1  IntegratorMethod=Forward Euler  FilterMethod=Forward Euler  ControllerParametersSource=internal  P=4  I=1  UseKiTs=off  D=0  N=100  UseFilter=on  TunerSelectOption=Transfer Function Based (PID Tuner App)  InitialConditionSource=internal  InitialConditionForIntegrator=0  InitialConditionForFilter=0  DifferentiatorICPrevScaledInput=0  ExternalReset=none  TrackingMode=off  Kt=1  LimitOutput=off  SatLimitsSource=internal  UpperSaturationLimit=inf  LowerSaturationLimit=-inf  LinearizeAsGain=on  AntiWindupMode=none  Kb=1  LimitIntegrator=off  UpperIntegratorSaturationLimit=inf  LowerIntegratorSaturationLimit=-inf  POutMin=[]  POutMax=[]  IOutMin=[]  IOutMax=[]  DOutMin=[]  DOutMax=[]  NOutMin=[]  NOutMax=[]  SumOutMin=[]  SumOutMax=[]  SaturationOutMin=[]  SaturationOutMax=[]  PParamMin=[]  PParamMax=[]  IParamMin=[]  IParamMax=[]  DParamMin=[]  DParamMax=[]  NParamMin=[]  NParamMax=[]  KbParamMin=[]  KbParamMax=[]  KtParamMin=[]  KtParamMax=[]  KbOutMin=[]  KbOutMax=[]  KtOutMin=[]  KtOutMax=[]  IntegratorOutMin=[]  IntegratorOutMax=[]  FilterOutMin=[]  FilterOutMax=[]  SumI1OutMin=[]  SumI1OutMax=[]  SumI2OutMin=[]  SumI2OutMax=[]  SumI3OutMin=[]  SumI3OutMax=[]  SumI4OutMin=[]  SumI4OutMax=[]  SumDOutMin=[]  SumDOutMax=[]  DifferentiatorOutMin=[]  DifferentiatorOutMax=[]  FilterDiffOutCoefMin=[]  FilterDiffOutCoefMax=[]  ReciprocalOutMin=[]  ReciprocalOutMax=[]  SumDenOutMin=[]  SumDenOutMax=[]  SumNumOutMin=[]  SumNumOutMax=[]  DivideOutMin=[]  DivideOutMax=[]  UdiffTsProdOutMin=[]  UdiffTsProdOutMax=[]  NTsProdOutMin=[]  NTsProdOutMax=[]  UintegralTsProdOutMin=[]  UintegralTsProdOutMax=[]  UngainTsProdOutMin=[]  UngainTsProdOutMax=[]  ClampingZeroOutDataTypeStr=Inherit: Inherit via back propagation  ClampingZeroOutMin=[]  ClampingZeroOutMax=[]  FilterDenConstantOutDataTypeStr=Inherit: Inherit via back propagation  FilterDenConstantOutMin=[]  FilterDenConstantOutMax=[]  PCopyOutDataTypeStr=Inherit: Inherit via back propagation  PCopyOutMin=[]  PCopyOutMax=[]  NCopyOutDataTypeStr=Inherit: Inherit via back propagation  NCopyOutMin=[]  NCopyOutMax=[]  IntegratorContinuousStateAttributes=''  IntegratorStateMustResolveToSignalObject=off  IntegratorRTWStateStorageClass=Auto  FilterContinuousStateAttributes=''  FilterStateMustResolveToSignalObject=off  FilterRTWStateStorageClass=Auto  ParallelPVariant=InternalParameters  IdealPVariant=Disabled  IVariant=Disabled  DVariant=Disabled  IntegratorVariant=Disabled  SatVariant=Disabled  AWVariant=Disabled  PCopyVariant=Disabled  TRVariant=Disabled  FdbkBlocksVariant=Forward  IdealPFdbkVariant=Disabled  SatFdbkVariant=Disabled  DerivativeFilterVariant=Disabled  NVariant=Disabled  NCopyVariant=Disabled_SignalSpec  FilterICVariant=Disabled  IntegratorICVariant=Disabled  ExternalResetVariant=Disabled  TRSumVariant=Passthrough  SumFdbkVariant=Disabled  SumVariant=Passthrough_P  TsampFilterVariant=InternalTs  TsampNgainVariant=Passthrough  TsampIntegralVariant=Disabled_SignalSpec  ExternalSaturationOutDataTypeStr=Inherit: Same as second input
  PID Controller5 : slpidlib/PID Controller  Controller=P  Form=Parallel  TimeDomain=Discrete-time  UseExternalTs=off  SampleTime=-1  IntegratorMethod=Forward Euler  FilterMethod=Forward Euler  ControllerParametersSource=internal  P=2  I=1  UseKiTs=off  D=0  N=100  UseFilter=on  TunerSelectOption=Transfer Function Based (PID Tuner App)  InitialConditionSource=internal  InitialConditionForIntegrator=0  InitialConditionForFilter=0  DifferentiatorICPrevScaledInput=0  ExternalReset=none  TrackingMode=off  Kt=1  LimitOutput=on  SatLimitsSource=internal  UpperSaturationLimit=50*pi/180  LowerSaturationLimit=-50*pi/180  LinearizeAsGain=on  AntiWindupMode=none  Kb=1  LimitIntegrator=off  UpperIntegratorSaturationLimit=inf  LowerIntegratorSaturationLimit=-inf  POutMin=[]  POutMax=[]  IOutMin=[]  IOutMax=[]  DOutMin=[]  DOutMax=[]  NOutMin=[]  NOutMax=[]  SumOutMin=[]  SumOutMax=[]  SaturationOutMin=[]  SaturationOutMax=[]  PParamMin=[]  PParamMax=[]  IParamMin=[]  IParamMax=[]  DParamMin=[]  DParamMax=[]  NParamMin=[]  NParamMax=[]  KbParamMin=[]  KbParamMax=[]  KtParamMin=[]  KtParamMax=[]  KbOutMin=[]  KbOutMax=[]  KtOutMin=[]  KtOutMax=[]  IntegratorOutMin=[]  IntegratorOutMax=[]  FilterOutMin=[]  FilterOutMax=[]  SumI1OutMin=[]  SumI1OutMax=[]  SumI2OutMin=[]  SumI2OutMax=[]  SumI3OutMin=[]  SumI3OutMax=[]  SumI4OutMin=[]  SumI4OutMax=[]  SumDOutMin=[]  SumDOutMax=[]  DifferentiatorOutMin=[]  DifferentiatorOutMax=[]  FilterDiffOutCoefMin=[]  FilterDiffOutCoefMax=[]  ReciprocalOutMin=[]  ReciprocalOutMax=[]  SumDenOutMin=[]  SumDenOutMax=[]  SumNumOutMin=[]  SumNumOutMax=[]  DivideOutMin=[]  DivideOutMax=[]  UdiffTsProdOutMin=[]  UdiffTsProdOutMax=[]  NTsProdOutMin=[]  NTsProdOutMax=[]  UintegralTsProdOutMin=[]  UintegralTsProdOutMax=[]  UngainTsProdOutMin=[]  UngainTsProdOutMax=[]  ClampingZeroOutDataTypeStr=Inherit: Inherit via back propagation  ClampingZeroOutMin=[]  ClampingZeroOutMax=[]  FilterDenConstantOutDataTypeStr=Inherit: Inherit via back propagation  FilterDenConstantOutMin=[]  FilterDenConstantOutMax=[]  PCopyOutDataTypeStr=Inherit: Inherit via back propagation  PCopyOutMin=[]  PCopyOutMax=[]  NCopyOutDataTypeStr=Inherit: Inherit via back propagation  NCopyOutMin=[]  NCopyOutMax=[]  IntegratorContinuousStateAttributes=''  IntegratorStateMustResolveToSignalObject=off  IntegratorRTWStateStorageClass=Auto  FilterContinuousStateAttributes=''  FilterStateMustResolveToSignalObject=off  FilterRTWStateStorageClass=Auto  ParallelPVariant=InternalParameters  IdealPVariant=Disabled  IVariant=Disabled  DVariant=Disabled  IntegratorVariant=Disabled  SatVariant=Enabled  AWVariant=Disabled  PCopyVariant=Disabled  TRVariant=Disabled  FdbkBlocksVariant=Forward  IdealPFdbkVariant=Disabled  SatFdbkVariant=Disabled  DerivativeFilterVariant=Disabled  NVariant=Disabled  NCopyVariant=Disabled_SignalSpec  FilterICVariant=Disabled  IntegratorICVariant=Disabled  ExternalResetVariant=Disabled  TRSumVariant=Passthrough  SumFdbkVariant=Disabled  SumVariant=Passthrough_P  TsampFilterVariant=InternalTs  TsampNgainVariant=Passthrough  TsampIntegralVariant=Disabled_SignalSpec  ExternalSaturationOutDataTypeStr=Inherit: Same as second input
  Rate Limiter1 : RateLimiter  RisingSlewLimit=40*pi/180  FallingSlewLimit=-40*pi/180  SampleTimeMode=inherited
  Rate Limiter2 : RateLimiter  RisingSlewLimit=40*pi/180  FallingSlewLimit=-40*pi/180  SampleTimeMode=inherited
  Saturation : Saturate  UpperLimit=20*pi/180  LowerLimit=-20*pi/180
  Saturation1 : Saturate  UpperLimit=20*pi/180  LowerLimit=-20*pi/180
  Sum{,1..5} (6 alike) : Sum  Inputs=|+-
  Unary Minus : UnaryMinus
  Unary Minus1 : UnaryMinus
  tau_Yaw : Outport
  tau_Pitch : Outport  Port=2
  tau_Roll : Outport  Port=3
  wires:
  PID Controller/1 -> tau_Yaw/1
  PID Controller2/1 -> Unary Minus1/1
  Sum/1 -> PID Controller1/1
  Ang rate/1 -> Demux/1
  Demux/2 -> Sum/2
  Unary Minus/1 -> tau_Pitch/1
  Sum1/1 -> PID Controller2/1
  Demux/1 -> Sum1/2
  Unary Minus1/1 -> tau_Roll/1
  Sum2/1 -> PID Controller3/1
  Sum3/1 -> PID Controller4/1
  ypr/1 -> Demux2/1
  Demux2/2 -> Sum2/2
  Demux2/3 -> Sum3/2
  Sum4/1 -> PID Controller/1
  Demux/3 -> Sum4/2
  Demux2/1 -> Sum5/2
  Sum5/1 -> Calculate minimum Turn/1(In1)
  Calculate minimum Turn/1(Out1) -> PID Controller5/1
  PID Controller1/1 -> Unary Minus/1
  des_roll/1 -> Rate Limiter1/1
  Rate Limiter1/1 -> Saturation/1
  Rate Limiter2/1 -> Saturation1/1
  des_yaw/1 -> Sum5/1
  Saturation/1 -> Sum3/1
  PID Controller3/1 -> Sum/1
  Saturation1/1 -> Sum2/1
  des_pitch/1 -> Rate Limiter2/1
  PID Controller4/1 -> Sum1/1
  PID Controller5/1 -> Sum4/1
